simulink model "lineal200"  (R2017a)
settings: Solver=VariableStepAuto  StartTime=0.0  StopTime=6000  RelTol=1e-3
values from neighbouring files (symbols this model uses):
  A = [-0.003401570000000  -0.000000016230000 ... (first row only)    [Lyglobal.m]
  B = [1;0]    [Lyglobal.m]
  C = [1 0]    [Lyglobal.m]
  D = 0    [Lyglobal.m]
  K = [8.997598430000000   0.008999983770000]    [Lyglobal.m]    (also in PDCtracking.m = [K k]; planta.m = acker(A,B,P))
settings Model: Creator=Dell  LastModifiedBy=Dell

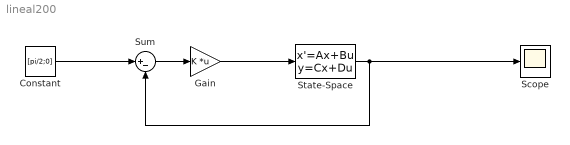
== system lineal200 ==
  Constant : Constant  Value=[pi/2;0]  VectorParams1D=off
  Gain : Gain  Gain=K  Multiplication=Matrix(K*u)
  Scope : Scope
  State-Space : StateSpace  A=A  B=B  C=C  D=D  X0=0
  Sum : Sum  Inputs=|+-
  wires:
  Sum/1 -> Gain/1
  Gain/1 -> State-Space/1
  Constant/1 -> Sum/1
  State-Space/1 -> Scope/1, Sum/2
